simulink subsystem "Trigger_Timer"  (R2022b)
settings: Solver=VariableStepAuto  StartTime=0.0  StopTime=10.0  RelTol=1e-3
settings Model: Creator=User  LastModifiedBy=User

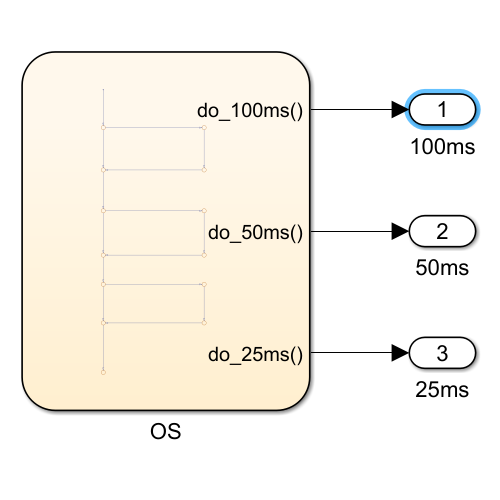
[thumbnail: Simulink's stored preview of the top-level diagram]
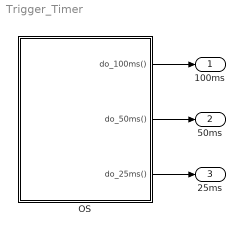
== system Trigger_Timer ==
  OS : Stateflow chart  TreatAsAtomicUnit=on
  100ms : Outport
  50ms : Outport  Port=2
  25ms : Outport  Port=3
  wires:
  OS/1(do_100ms()) -> 100ms/1
  OS/2(do_50ms()) -> 50ms/1
  OS/3(do_25ms()) -> 25ms/1

== stateflow chart Trigger_Timer/OS ==
  (default) -> (junction 2)
  (junction 2) -> (junction 10) [order 1] : [rem(time_en3,100) == 0]
  (junction 2) -> (junction 4) [order 2]
  (junction 10) -> (junction 12) : {
      |
      |   do_100ms
      | }
  (junction 12) -> (junction 4)
  (junction 4) -> (junction 6)
  (junction 6) -> (junction 16) [order 1] : [rem(time_en3,50) == 0]
  (junction 6) -> (junction 21) [order 2]
  (junction 16) -> (junction 19) : {
      |
      |   do_50ms
      | }
  (junction 19) -> (junction 21)
  (junction 21) -> (junction 23)
  (junction 23) -> (junction 32) [order 1] : [rem(time_en3,25) == 0]
  (junction 23) -> (junction 33) [order 2]
  (junction 32) -> (junction 30) : {
      |
      |   do_25ms
      | }
  (junction 30) -> (junction 33)
  (junction 33) -> (junction 36) : {
      | time_en3 = rem(time_en3, 200);
      | time_en3 = time_en3 +1;
      | }
  data: time_en3 local int32 =int32(0)
  events: do_100ms output FUNCTION_CALL_EVENT; do_50ms output FUNCTION_CALL_EVENT; do_25ms output FUNCTION_CALL_EVENT
